simulink model "Zarc"  (R2012b)
settings: Solver=ode45  StartTime=0.0  StopTime=10.0  RelTol=1e-3
settings Model: Creator=sz609516  LastModifiedBy=sz609516
settings DataIOCC: SignalLoggingSaveFormat=ModelDataLogs
settings DebuggingCC: FcnCallInpInsideContextMsg=EnableAllAsWarning
settings GRTTargetCC: CombineOutputUpdateFcns=off  GRTInterface=on

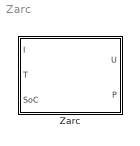
== system Zarc ==
  Zarc : Subsystem

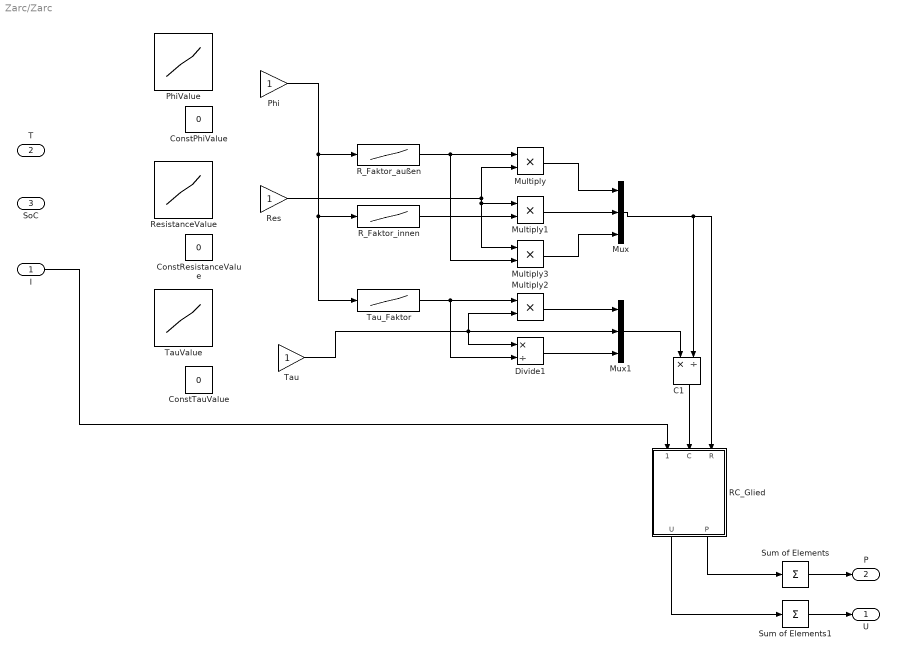
== system Zarc/Zarc ==
  I : Inport
  T : Inport  Port=2
  SoC : Inport  Port=3
  C1 : Product  Inputs=*/
  ConstPhiValue : Constant  Value=0
  ConstResistanceValue : Constant  Value=0
  ConstTauValue : Constant  Value=0
  Divide1 : Product  Inputs=*/
  Multiply{,1..3} (4 alike) : Product  Inputs=**
  Mux : Mux  Inputs=3
  Mux1 : Mux  Inputs=3
  Phi : Gain
  PhiValue : Lookup_n-D  Table=[1,2,3;4,5,6;7,8,9]  ExtrapMethod=Clip  RndMeth=Simplest  InputSameDT=on
  RC_Glied : Subsystem
  R_Faktor_außen : Lookup  InputValues="[ 0.4         0.5         0.6         0.7         0.8         0.9        0.92        0.94        0.96        0.98           1 ]"  Table="[ 0.28084     0.26535      0.2446     0.21576     0.17431     0.11057    0.093487    0.074352     0.05276    0.028198           0 ]"  SaturateOnIntegerOverflow=on
  R_Faktor_innen : Lookup  InputValues="[ 0.4         0.5         0.6         0.7         0.8         0.9        0.92        0.94        0.96        0.98           1 ]"  Table="[ 0.39633     0.44284     0.49461     0.55903     0.64641     0.77687      0.8115      0.8502     0.89378     0.94327           1 ]"  SaturateOnIntegerOverflow=on
  Res : Gain
  ResistanceValue : Lookup_n-D  Table=[1,2,3;4,5,6;7,8,9]  ExtrapMethod=Clip  RndMeth=Simplest  InputSameDT=on
  Sum of Elements : Sum  Inputs=+
  Sum of Elements1 : Sum  Inputs=+
  Tau : Gain
  TauValue : Lookup_n-D  Table=[1,2,3;4,5,6;7,8,9]  ExtrapMethod=Clip  RndMeth=Simplest  InputSameDT=on
  Tau_Faktor : Lookup  InputValues="[0.4         0.5         0.6         0.7         0.8         0.9        0.92        0.94        0.96        0.98           1]"  Table=|  SaturateOnIntegerOverflow=on
      | [39.9742      21.8364      13.6186      9.23106      6.58365      4.83194       4.5502      4.28597      4.03746      3.80306      3.58133
      | ]
  U : Outport
  P : Outport  Port=2
  wires:
  Mux/1 -> C1/2, RC_Glied/3(R)
  Mux1/1 -> C1/1
  Tau_Faktor/1 -> Divide1/2, Multiply2/1
  Divide1/1 -> Mux1/3
  Multiply2/1 -> Mux1/1
  Multiply3/1 -> Mux/3
  Multiply1/1 -> Mux/2
  Multiply/1 -> Mux/1
  R_Faktor_innen/1 -> Multiply1/2
  R_Faktor_außen/1 -> Multiply3/2, Multiply/1
  I/1 -> RC_Glied/1(I_charge_bez)
  C1/1 -> RC_Glied/2(C)
  RC_Glied/2(P) -> Sum of Elements/1
  RC_Glied/1(U) -> Sum of Elements1/1
  Sum of Elements1/1 -> U/1
  Sum of Elements/1 -> P/1
  Phi/1 -> R_Faktor_außen/1, R_Faktor_innen/1, Tau_Faktor/1
  Tau/1 -> Mux1/2, Multiply2/2, Divide1/1
  Res/1 -> Multiply/2, Multiply1/1, Multiply3/1

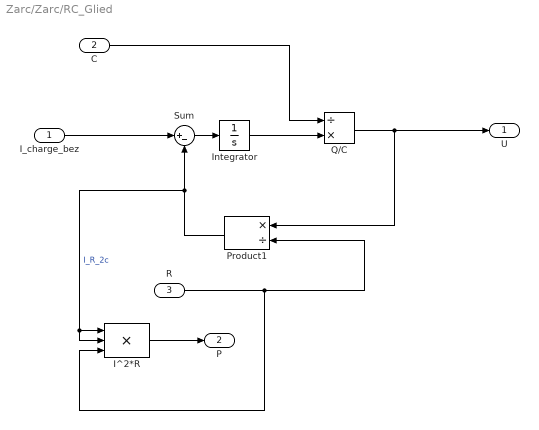
== system Zarc/Zarc/RC_Glied ==
  I_charge_bez : Inport
  C : Inport  Port=2
  R : Inport  Port=3
  I^2*R : Product  Inputs=3  SaturateOnIntegerOverflow=on  OutDataTypeStr=Inherit: Same as first input
  Integrator : Integrator
  Product1 : Product  Inputs=*/  SaturateOnIntegerOverflow=on  OutDataTypeStr=Inherit: Same as first input
  Q/C : Product  Inputs=/*
  Sum : Sum  Inputs=|+-  SaturateOnIntegerOverflow=on  InputSameDT=on  OutDataTypeStr=Inherit: Same as first input
  U : Outport
  P : Outport  Port=2
  wires:
  Integrator/1 -> Q/C/2
  Q/C/1 -> Product1/1, U/1
  Sum/1 -> Integrator/1
  I_charge_bez/1 -> Sum/1
  Product1/1 -> Sum/2, I^2*R/1, I^2*R/2  "I_R_2c"
  R/1 -> Product1/2, I^2*R/3
  C/1 -> Q/C/1
  I^2*R/1 -> P/1
